simulink model "SB3_subsys_todo"  (R2024b)
settings: Solver=FixedStepDiscrete  StartTime=0.0  StopTime=5  FixedStep=0.05  RelTol=1e-3
settings Model: Creator=admin  LastModifiedBy=admin

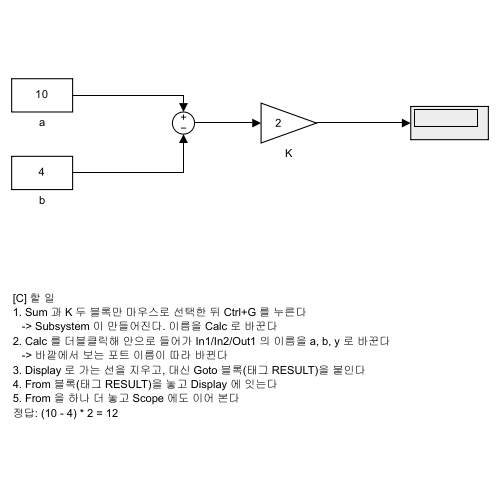
[thumbnail: Simulink's stored preview of the top-level diagram]
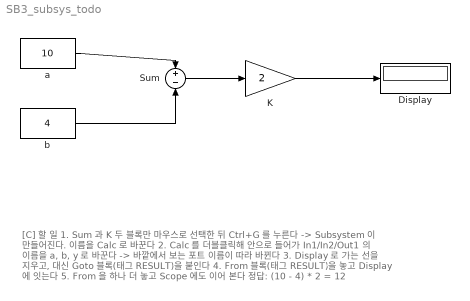
== system SB3_subsys_todo ==
  note: [C] 할 일
      | 1. Sum 과 K 두 블록만 마우스로 선택한 뒤 Ctrl+G 를 누른다
      |    -> Subsystem 이 만들어진다. 이름을 Calc 로 바꾼다
      | 2. Calc 를 더블클릭해 안으로 들어가 In1/In2/Out1 의 이름을 a, b, y 로 바꾼다
      |    -> 바깥에서 보는 포트 이름이 따라 바뀐다
      | 3. Display 로 가는 선을 지우고, 대신 Goto 블록(태그 RESULT)을 붙인다
      | 4. From 블록(태그 RESULT)을 놓고 Display 에 잇는다
      | 5. From 을 하나 더 놓고 Scope 에도 이어 본다
      | 정답: (10 - 4) * 2 = 12
  Display : Display
  K : Gain  Gain=2
  Sum : Sum  Inputs=+-
  a : Constant  Value=10
  b : Constant  Value=4
  wires:
  a/1 -> Sum/1
  b/1 -> Sum/2
  Sum/1 -> K/1
  K/1 -> Display/1
